simulink model "q_three_woaw"  (R2019b)
settings: Solver=VariableStepAuto  StartTime=0.0  StopTime=1  RelTol=1e-3
values from neighbouring files (symbols this model uses):
  A1 = [(-Ra/La) ((-ka*ia)/La); ((ka*ia)/J) (-B/J)]    [ex2.m]    (also in ex3.m = [(-Ra/La) ((-ka*ia)/La); (ka*ia)/J -(B/J)])
  B1 = [(1/La) 0; 0 (-1/J)]    [ex2.m]    (also in ex3.m)
  C1 = [1 0;0 1]    [ex2.m]    (also in ex3.m)
  D1 = [0 0;0 0]    [ex2.m]    (also in ex3.m)
  kq2 = k    [ex3.m]
  kq3 = place(A3, B3, p3)    [ex3.m]
settings Model: Creator=rafek  LastModifiedBy=rafek

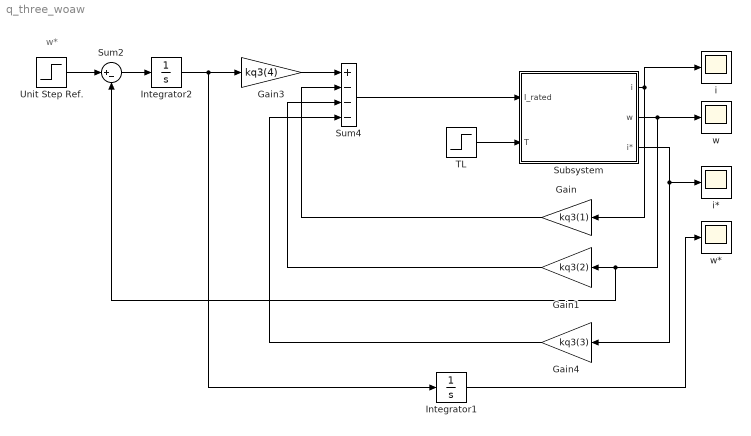
== system q_three_woaw ==
  note: w*
  Gain : Gain  Gain=kq3(1)
  Gain1 : Gain  Gain=kq3(2)
  Gain3 : Gain  Gain=kq3(4)
  Gain4 : Gain  Gain=kq3(3)
  Integrator1 : Integrator
  Integrator2 : Integrator
  Subsystem : Subsystem
  Sum2 : Sum  Inputs=|+-
  Sum4 : Sum  Inputs=+---
  TL : Step  Time=0  After=0  SampleTime=0
  Unit Step Ref. : Step  Time=0  SampleTime=0
  i : Scope
  i* : Scope
  w : Scope
  w* : Scope
  wires:
  Integrator1/1 -> w*/1
  Sum4/1 -> Subsystem/1(I_rated)
  Gain3/1 -> Sum4/1
  Subsystem/3(i*) -> Gain4/1, i*/1
  Gain1/1 -> Sum4/3
  Sum2/1 -> Integrator2/1
  Subsystem/1(i) -> Gain/1, i/1
  Gain4/1 -> Sum4/4
  TL/1 -> Subsystem/2(T)
  Subsystem/2(w) -> Sum2/2, Gain1/1, w/1
  Unit Step Ref./1 -> Sum2/1
  Gain/1 -> Sum4/2
  Integrator2/1 -> Integrator1/1, Gain3/1

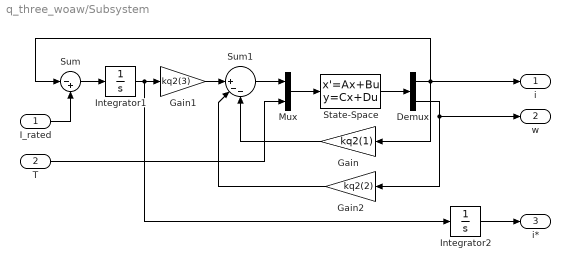
== system q_three_woaw/Subsystem ==
  I_rated : Inport
  T : Inport  Port=2
  Demux : Demux  Outputs=2
  Gain : Gain  Gain=kq2(1)
  Gain1 : Gain  Gain=kq2(3)
  Gain2 : Gain  Gain=kq2(2)
  Integrator1 : Integrator
  Integrator2 : Integrator
  Mux : Mux  Inputs=2
  State-Space : StateSpace  A=A1  B=B1  C=C1  D=D1  InitialCondition=0
  Sum : Sum  Inputs=|-+
  Sum1 : Sum  Inputs=||+--
  i : Outport  VectorParamsAs1DForOutWhenUnconnected=off
  w : Outport  Port=2  VectorParamsAs1DForOutWhenUnconnected=off
  i* : Outport  Port=3  VectorParamsAs1DForOutWhenUnconnected=off
  wires:
  T/1 -> Mux/2
  Mux/1 -> State-Space/1
  Gain2/1 -> Sum1/2
  Gain1/1 -> Sum1/1
  Demux/2 -> Gain2/1, w/1
  Sum1/1 -> Mux/1
  I_rated/1 -> Sum/2
  Demux/1 -> Sum/1, i/1, Gain/1
  State-Space/1 -> Demux/1
  Gain/1 -> Sum1/3
  Sum/1 -> Integrator1/1
  Integrator1/1 -> Integrator2/1, Gain1/1
  Integrator2/1 -> i*/1
